simulink model "ric_paralelo"  (R2015a)
settings: Solver=ode45  StartTime=0.0  StopTime=5  RelTol=1e-6  AbsTol=1e-6
undefined symbols (not defined in the file): C, i, L, R
libraries: fl_lib x7, nesl_utility x4
settings Model: Creator=11802972  LastModifiedBy=11802972

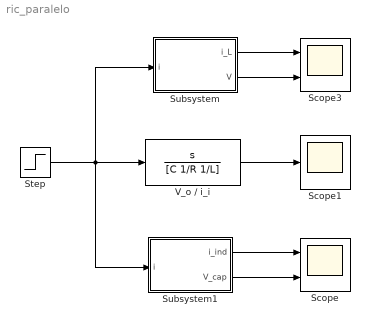
== system ric_paralelo ==
  Scope : Scope  NumInputPorts=2
      settings: YMin=-5~-5  YMax=5~5
  Scope1 : Scope
  Scope3 : Scope  NumInputPorts=2
      settings: YMin=-5~-5  YMax=5~5  SaveName=ScopeData3
  Step : Step  After=i  SampleTime=0
  Subsystem : Subsystem
  Subsystem1 : Subsystem
  V_o / i_i : TransferFcn  Numerator=[1 0]  Denominator=[C 1/R 1/L]
  wires:
  Step/1 -> Subsystem/1(i), V_o / i_i/1, Subsystem1/1(i)
  Subsystem1/1(i_ind) -> Scope/1
  Subsystem1/2(V_cap) -> Scope/2
  V_o / i_i/1 -> Scope1/1
  Subsystem/1(i_L) -> Scope3/1
  Subsystem/2(V) -> Scope3/2

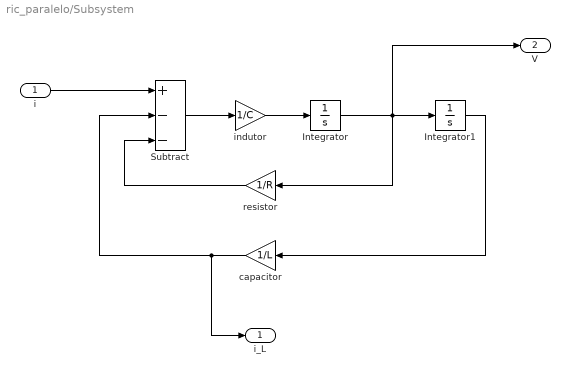
== system ric_paralelo/Subsystem ==
  i : Inport
  Integrator : Integrator
  Integrator1 : Integrator
  Subtract : Sum  Inputs=+--
  capacitor : Gain  Gain=1/L
  indutor : Gain  Gain=1/C
  resistor : Gain  Gain=1/R
  i_L : Outport
  V : Outport  Port=2
  wires:
  Subtract/1 -> indutor/1
  i/1 -> Subtract/1
  resistor/1 -> Subtract/3
  Integrator/1 -> V/1, Integrator1/1, resistor/1
  capacitor/1 -> i_L/1, Subtract/2
  Integrator1/1 -> capacitor/1
  indutor/1 -> Integrator/1

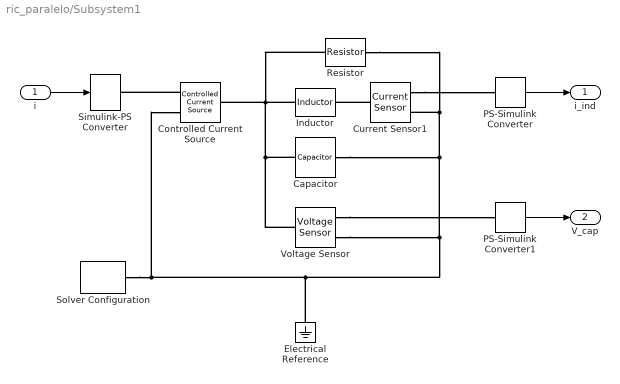
== system ric_paralelo/Subsystem1 ==
  i : Inport
  Capacitor : fl_lib/Electrical/Electrical Elements/Capacitor  c=C F  r=0 Ohm  g=0 1/Ohm  i_specify=off  i_priority=High  i=0 A  v_specify=off  v_priority=High  v=0 V  vc_specify=off  vc_priority=High  vc=0 V
  Controlled Current Source : fl_lib/Electrical/Electrical Sources/Controlled Current Source
  Current Sensor1 : fl_lib/Electrical/Electrical Sensors/Current Sensor
  Electrical Reference : fl_lib/Electrical/Electrical Elements/Electrical Reference
  Inductor : fl_lib/Electrical/Electrical Elements/Inductor  l=L H  r=0 Ohm  g=0 1/Ohm  i_specify=off  i_priority=High  i=0 A  v_specify=off  v_priority=High  v=0 V  i_L_specify=off  i_L_priority=High  i_L=0 A
  PS-Simulink Converter : nesl_utility/PS-Simulink Converter  PhysicalDomain=network_engine_domain  SubClassName=ps_output  LeftPortType=input  RightPortType=output  PseudoPeriodic=off  Frequencies=[]  Unit=1  AffineConversion=off
  PS-Simulink Converter1 : nesl_utility/PS-Simulink Converter  PhysicalDomain=network_engine_domain  SubClassName=ps_output  LeftPortType=input  RightPortType=output  PseudoPeriodic=off  Frequencies=[]  Unit=1  AffineConversion=off
  Resistor : fl_lib/Electrical/Electrical Elements/Resistor  R=R Ohm  i_specify=off  i_priority=High  i=0 A  v_specify=off  v_priority=High  v=0 V
  Simulink-PS Converter : nesl_utility/Simulink-PS Converter  PhysicalDomain=network_engine_domain  SubClassName=ps_input  LeftPortType=input  RightPortType=output  PseudoPeriodic=off  Frequencies=[]  NoiseDistribution=none  NoiseParameters=[]  Unit=1  AffineConversion=off  InputFiltering=off  SimscapeFilterOrder=1  InputFilterTimeConstant=0.001  UdotUserProvided=1
  Solver Configuration : nesl_utility/Solver Configuration  PhysicalDomain=network_engine_domain  SubClassName=solver  LeftPortType=input  RightPortType=generic  Accelerate=off  Tones=[]  Harmonics=[]  SimulateNoise=off  Profile=off  UseLocalSampling=off  EnableSwitchedLinearOptims=on  FrequencyDomain=off  UseCCode=off  RelTol=0.001  AbsTol=1e-06  MinStep=1e-09  ToWorkspace=off  RevertToSquareIcSolve=off  NumHomotopyIterations=100  DoDC=off  ResidualTolerance=1e-06  UseLocalSolver=off  LocalSolverChoice=NE_BACKWARD_EULER_ADVANCER  LocalSolverSampleTime=0.001  DoFixedCost=off  MaxNonlinIter=3  MaxModeIter=2  LinearAlgebra=Sparse  DelaysMemoryBudget=1024  AutomaticFiltering=on  FilteringTimeConstant=0.001
  Voltage Sensor : fl_lib/Electrical/Electrical Sensors/Voltage Sensor
  i_ind : Outport
  V_cap : Outport  Port=2
  wires:
  PS-Simulink Converter/1 -> i_ind/1
  i/1 -> Simulink-PS Converter/1
  PS-Simulink Converter1/1 -> V_cap/1
  connections:
  Controlled Current Source/RConn1 -- Simulink-PS Converter/RConn1
  Resistor/LConn1 -- Voltage Sensor/LConn1 -- Capacitor/LConn1 -- Inductor/LConn1 -- Controlled Current Source/LConn1
  Resistor/RConn1 -- Electrical Reference/LConn1 -- Solver Configuration/RConn1 -- Controlled Current Source/RConn2 -- Voltage Sensor/RConn2 -- Capacitor/RConn1 -- Current Sensor1/RConn2
  Current Sensor1/LConn1 -- Inductor/RConn1
  Current Sensor1/RConn1 -- PS-Simulink Converter/LConn1
  Voltage Sensor/RConn1 -- PS-Simulink Converter1/LConn1
